simulink library "socmemlib"  (R2021a)
settings: Solver=VariableStepAuto  StartTime=0.0  StopTime=10.0  RelTol=1e-3
PreLoadFcn:
  | soc.internal.HWSWMessageTypeDef();
  | hsb.blkcb2.defineTypes;
undefined symbols (not defined in the file or in its folder): BurstRequest2BusObj, gcbh, hsb, m, ReadAccessBusObj, rearb, RegA, sendFifoFreeMsg, soc, WriteAccessBusObj
libraries: socmemlib_internal x59, priv_hsblib_beta2 x34, socsharedlib_internal x2, socqueuelib_internal x1, simulink x1
(part 1 of 5)
settings Model: Creator=The MathWorks, Inc.  LastModifiedBy=jchevali
settings SolverCC: AlgebraicLoopSolver=TrustRegion
settings DataIOCC: ReturnWorkspaceOutputs=off
settings DebuggingCC: PregeneratedLibrarySubsystemCodeDiagnostic=none  SFMachineParentedDataDiag=warning  ArithmeticOperatorsInVariantConditions=warning
settings SFSimCC: SimUseLocalCustomCode=off
settings RTWCC: RTWUseLocalCustomCode=off

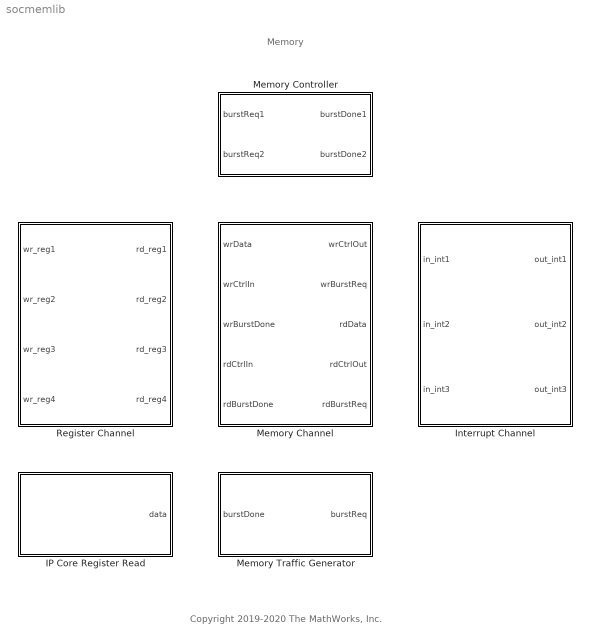
== system socmemlib ==
  note: Memory
  note: Copyright 2019-2020 The MathWorks, Inc.
  IP Core Register Read : Subsystem  InitFcn=soc.blkcb.IPCoreRegisterReadCb('InitFcnCb',gcbh);  mask(IP Core Register Read){RegisterName=RegA, OutDataTypeStr=uint16, OutputVectorSize=1, SampleTime=-1}
      mask prompts: RegisterName "Register name:"; OutDataTypeStr "Output data type:"; OutputVectorSize "Output vector size:"; SampleTime "Sample time:"
      mask help:
      | Read data from a memory-mapped register of a hardware logic IP core.
      |
      | The block interfaces with a Register Write block and outputs the read data.
      |
      | Set the Output data type and Output vector size parameters to match the equivalents in the register being read.
      mask init:
      | soc.blkcb.IPCoreRegisterReadCb('MaskInitFcn',gcbh);
      mask Help: eval('soc.internal.helpview(''soc_ipcoreregisterread'')')
      mask TypeOptions RegisterName: Variant/SIM/Wireless Read/RegisterName
      mask Callback RegisterName: soc.blkcb.IPCoreRegisterReadCb('RegisterNameCb',gcbh);
      mask TypeOptions SampleTime: Variant/SIM/Wireless Read/SampleTime
      mask DialogControl DescGroupVar Prompt: IP Core Register Read
      mask Display:
      | color('black');
      | text(0.5, 0.85, 'RegA','horizontalAlignment','center','texmode','off');
  Interrupt Channel : Subsystem  LoadFcn=soc.blkcb.InterruptChannelCb('LoadFcn', gcbh);  InitFcn=soc.blkcb.InterruptChannelCb('InitFcn', gcbh);  mask(Interrupt Channel){InterruptTable={'interrupt1','Rising edge','1';'interrupt2','Rising edge','2';'interrupt3','Rising edge','3'}, InterruptProcessingTime=100e-6, IntTableNames={'interrupt1' 'interrupt2' 'interrupt3' }, IntTableTriggers={'Rising edge' 'Rising edge' 'Rising edge' }, NumInterrupts=3, IntTableDirty=0}
      mask prompts: InterruptTable "Interrupts"; InterruptProcessingTime "Interrupt processing time:"; IntTableNames "(int table names)"; IntTableTriggers "(int table triggers)"; NumInterrupts "(num interrupts)"; IntTableDirty "(int table dirty)"
      mask help:
      | Model interrupts from FPGA to processor.
      |
      | Each pair of input and output ports with the same name represent an interrupt. On the FPGA side (HW) each input interfaces with a boolean signal from the FPGA, or an event from an Event Source or Memory Channel blocks. On the processor side (SW) each output connects to a Task Manager event input port.
      |
      | Add or remove interrupts by using the New and Delete buttons, respectively. To change the priority of interrupts, arrange their order using the Move Up and Move Down buttons. Change the Name and Trigger Type of an interrupt by editing the value in the table. Set the interrupt Trigger Type to Rising Edge if the interrupt is coming from FPGA logic. Set the interrupt Trigger Type to SoC event if the interrupt is coming from Event Source block or Memory Channel block.
      mask init:
      | soc.blkcb.InterruptChannelCb('MaskInitFcn', gcbh, gcs);
      settings: PreSaveFcn=soc.blkcb.InterruptChannelCb('PreSaveFcn', gcbh);  PreCopyFcn=soc.blkcb.InterruptChannelCb('PreCopyFcn', gcbh);
      mask Help: eval('soc.internal.helpview(''soc_interruptchannel'')')
      mask Callback InterruptTable: soc.blkcb.InterruptChannelCb('EditTableRowCb', gcbh);
      mask Callback IntTableDirty: soc.blkcb.InterruptChannelCb('ResetTableCb', gcbh);
      mask DialogControl DescGroupVar Prompt: Interrupt Channel
      mask DialogControl AddRow Prompt: New
      mask DialogControl AddRow Callback: soc.blkcb.InterruptChannelCb('AddTableRowCb', gcbh);
      mask DialogControl MoveUpRow Prompt: Move Up
      mask DialogControl MoveUpRow Callback: soc.blkcb.InterruptChannelCb('ShiftTableRowUpCb', gcbh);
      mask DialogControl MoveDownRow Prompt: Move Down
      mask DialogControl MoveDownRow Callback: soc.blkcb.InterruptChannelCb('ShiftTableRowDownCb', gcbh);
      mask DialogControl DeleteRow Prompt: Delete
      mask DialogControl DeleteRow Callback: soc.blkcb.InterruptChannelCb('DeleteTableRowCb', gcbh);
      mask DialogControl AdvancedParametersPanel Prompt: Advanced
      mask DialogControl TableSupportParameterGroup Prompt: (Parameters - hidden)
      mask Display:
      | text(0.02,0.95,'{\bfHW}','horizontalAlignment','left', 'texmode','on');
      | text(0.98,0.95,'{\bfSW}','horizontalAlignment','right','texmode','on');
      | port_label('input', 1, 'interrupt1');
      | port_label('input', 2, 'interrupt2');
      | port_label('input', 3, 'interrupt3');
      | 
      | port_label('output', 1, 'interrupt1');
      | port_label('output', 2, 'interrupt2');
      | port_label('output', 3, 'interrupt3');
  Memory Channel : Subsystem  InstantiateOnLoad=on  LoadFcn=hsb.blkcb2.MemoryChannelCbV1('LoadFcn',gcbh);  InitFcn=hsb.blkcb2.MemoryChannelCbV1('InitFcn',gcbh);  mask(Memory Channel){ChannelType=AXI4-Stream FIFO, MRBufferSize=4096, MRNumBuffers=8, BurstLengthWriterChIf=256, BurstLengthReaderChIf=256, UseValuesFromTargetHardwareResources=on, ReaderWriterUseSameValues=on, FIFODepthWriter=8, FIFODepthReader=8, FIFOAFullDepthWriter=6, FIFOAFullDepthReader=6, ICClockFrequencyWriter=100, ICClockFrequencyReader=100, ICDataWidthWriter=64, ICDataWidthReader=64, ChDimensionsWriterChIf=1024, ChTypeWriterChIf=uint32, ChFrameSampleTimeWriterChIf=1, ChBitPackedWriterChIf=off, OutSigSpecMatchesInSigSpec=on, ChDimensionsReaderChIf=1024, ChTypeWithInhReaderChIf=uint32, ChFrameSampleTimeReaderChIf=1, ChBitPackedReaderChIf=off, InsertInactivePixelClocksReaderChIf=off, FrameSizeReaderChIf=160x120p, ProtocolWriter=AXI4-Stream, ProtocolReader=AXI4-Stream, ChTypeReaderChIf=uint32, LastTargetBoard=None, Beta2Compatible=off, MRRegionSize=32768, DiagnosticLevel=No debug, MRBaseAddress=hex2dec('00010000'), UseTargetGlobalValues=off, InterruptHandlingTimeWriterChIf=10e-6, BufferEventIDWriterChIf=NOT_USED, BufferLengthReaderChIf=NOT_USED, InterruptHandlingTimeReaderChIf=10e-6, BufferEventIDReaderChIf=NOT_USED}
      mask prompts: ChannelType "soc:ui:ChannelTypePR"; MRBufferSize "soc:ui:MRBufferSizePR"; MRNumBuffers "soc:ui:MRNumBuffersPR"; BurstLengthWriterChIf "Writer:"; BurstLengthReaderChIf "Reader:"; UseValuesFromTargetHardwareResources "soc:ui:UseValuesFromTargetHardwareResourcesPR"; ReaderWriterUseSameValues "soc:ui:ReaderWriterUseSameValuesPR"; FIFODepthWriter "Writer:"; FIFODepthReader "Reader:"; FIFOAFullDepthWriter "Writer:"; FIFOAFullDepthReader "Reader:"; ICClockFrequencyWriter "Writer:"; ICClockFrequencyReader "Reader:"; ICDataWidthWriter "Writer:"; ICDataWidthReader "Reader:"; ChDimensionsWriterChIf "soc:ui:ChDimensionsPR"; ChTypeWriterChIf "soc:ui:ChTypePR"; ChFrameSampleTimeWriterChIf "soc:ui:ChFrameSampleTimePR"; ChBitPackedWriterChIf "soc:ui:ChBitPackedPR"; OutSigSpecMatchesInSigSpec "soc:ui:OutSigSpecMatchesInSigSpecPR"; ChDimensionsReaderChIf "soc:ui:ChDimensionsPR"; ChTypeWithInhReaderChIf "soc:ui:ChTypeWithInhPR"; ChFrameSampleTimeReaderChIf "soc:ui:ChFrameSampleTimePR"; ChBitPackedReaderChIf "soc:ui:ChBitPackedPR"; InsertInactivePixelClocksReaderChIf "soc:ui:InsertInactivePixelClocksPR"; FrameSizeReaderChIf "soc:ui:FrameSizePR"; ProtocolWriter "soc:ui:ProtocolPR"; ProtocolReader "soc:ui:ProtocolPR"; ChTypeReaderChIf "soc:ui:ChTypePR"; LastTargetBoard "soc:ui:LastTargetBoardPR"; Beta2Compatible "soc:ui:Beta2CompatiblePR"; MRRegionSize "soc:ui:MRRegionSizePR"; DiagnosticLevel "soc:ui:DiagnosticLevelPR"; MRBaseAddress "soc:ui:MRBaseAddressPR"; UseTargetGlobalValues "soc:ui:UseTargetGlobalValuesPR"; InterruptHandlingTimeWriterChIf "soc:ui:InterruptHandlingTimePR"; BufferEventIDWriterChIf "soc:ui:BufferEventIDPR"; BufferLengthReaderChIf "soc:ui:BufferLengthPR"; InterruptHandlingTimeReaderChIf "soc:ui:InterruptHandlingTimePR"; BufferEventIDReaderChIf "soc:ui:BufferEventIDPR"
      mask help:
      | Model memory accesses as read and write bursts.
      |
      | Data, CtrlIn and CtrlOut ports read and write data. burstReq and burstDone ports manage requests to the Memory Controller.
      |
      | Burst length, Bandwidth, FIFO depth and other parameters can be changed in the Advanced section. In the Performance tab, metrics can be visualized after running a simulation.
      mask init:
      | blkH = gcbh;
      | blkDP = hsb.blkcb2.MemoryChannelCbV1('MaskInitFcnGetDerivedInfo',blkH);
      | hsb.blkcb2.MemoryChannelCbV1('MaskInitFcnSetDerivedInfo',blkH);
      settings: CopyFcn=hsb.blkcb2.MemoryChannelCbV1('CopyFcn',gcbh);  DeleteFcn=hsb.blkcb2.MemoryChannelCbV1('DeleteFcn',gcbh);  UndoDeleteFcn=hsb.blkcb2.MemoryChannelCbV1('UndoDeleteFcn',gcbh);  PreSaveFcn=hsb.blkcb2.MemoryChannelCbV1('PreSaveFcn',gcbh);  PortSchema="{\"entries\":[{\"content\":{\"connectorPositions\":[{\"content\":{\"connectorId\":\"In1\",\"location\":{\"content\":{\"denominator\":4,\"numerator\":1},\"type\":\"ConnectorPlacement.Fraction\"}},\"type\":\"ConnectorPlacement.RectBoundaryConnectorPosition\",\"uuid\":\"4c70ce42-7c73-4e93-ae07-074aaf1a9a86\"},{\"content\":{\"connectorId\":\"In2\",\"location\":{\"content\":{\"denominator\":4,\"numerator\":2},\"type\":\"ConnectorPlacement.Fraction\"}},\"type\":\"ConnectorPlacement.RectBoundaryConnectorPosition\",\"uuid\":\"b2362bf4-8aa6-405f-91d1-9667f6c9d620\"},{\"content\":{\"connectorId\":\"Out2\",\"location\":{\"content\":{\"denominator\":6,\"numerator\":1},\"type\":\"ConnectorPlacement.Fraction\"},\"rectSide\":\"TOP\"},\"type\":\"ConnectorPlacement.RectBoundaryConnectorPosition\",\"uuid\":\"7d756ea6-45bf-43e7-b630-38b77ea0e8f5\"},{\"content\":{\"connectorId\":\"Out1\",\"location\":{\"content\":{\"denominator\":4,\"numerator\":3},\"type\":\"ConnectorPlacement.Fraction\"}},\"type\":\"ConnectorPlacement.RectBoundaryConnectorPosition\",\"uuid\":\"c5018aec-8900-4eff-a24e-86b98029d217\"},{\"content\":{\"connectorId\":\"Out3\",\"location\":{\"content\":{\"denominator\":4,\"numerator\":1},\"type\":\"ConnectorPlacement.Fraction\"},\"rectSide\":\"RIGHT\"},\"type\":\"ConnectorPlacement.RectBoundaryConnectorPosition\",\"uuid\":\"77d0fbb5-db66-42ea-8c77-7d5ac595f097\"},{\"content\":{\"connectorId\":\"In3\",\"location\":{\"content\":{\"denominator\":6,\"numerator\":2},\"type\":\"ConnectorPlacement.Fraction\"},\"rectSide\":\"TOP\"},\"type\":\"ConnectorPlacement.RectBoundaryConnectorPosition\",\"uuid\":\"87aa62bc-c370-4d37-a540-9ec95a64357e\"},{\"content\":{\"connectorId\":\"<spacer>\",\"location\":{\"content\":{\"denominator\":4,\"numerator\":4},\"type\":\"ConnectorPlacement.Fraction\"}},\"type\":\"ConnectorPlacement.RectBoundaryConnectorPosition\",\"uuid\":\"c67822ed-a56d-48ae-950d-1631e90369e8\"},{\"content\":{\"connectorId\":\"<spacer>\",\"location\":{\"content\":{\"denominator\":6,\"numerator\":3},\"type\":\"ConnectorPlacement.Fraction\"},\"rectSide\":\"TOP\"},\"type\":\"ConnectorPlacement.RectBoundaryConnectorPosition\",\"uuid\":\"003a3c20-1809-4b81-91dd-db381fae4435\"},{\"content\":{\"connectorId\":\"Out4\",\"location\":{\"content\":{\"denominator\":4,\"numerator\":2},\"type\":\"ConnectorPlacement.Fraction\"},\"rectSide\":\"RIGHT\"},\"type\":\"ConnectorPlacement.RectBoundaryConnectorPosition\",\"uuid\":\"b50bd39a-3039-4a60-9d5f-00df12594061\"},{\"content\":{\"connectorId\":\"In4\",\"location\":{\"content\":{\"denominator\":4,\"numerator\":3},\"type\":\"ConnectorPlacement.Fraction\"},\"rectSide\":\"RIGHT\"},\"type\":\"ConnectorPlacement.RectBoundaryConnectorPosition\",\"uuid\":\"5399552b-01fb-4fbb-8d3f-cf2158907ef0\"},{\"content\":{\"connectorId\":\"Out5\",\"location\":{\"content\":{\"denominator\":6,\"numerator\":4},\"type\":\"ConnectorPlacement.Fraction\"},\"rectSide\":\"TOP\"},\"type\":\"ConnectorPlacement.RectBoundaryConnectorPosition\",\"uuid\":\"a671590f-6554-46f1-a67a-ef24abb9d788\"},{\"content\":{\"connectorId\":\"In5\",\"location\":{\"content\":{\"denominator\":6,\"numerator\":5},\"type\":\"ConnectorPlacement.Fraction\"},\"rectSide\":\"TOP\"},\"type\":\"ConnectorPlacement.RectBoundaryConnectorPosition\",\"uuid\":\"e91528d7-90f4-49f4-ae0e-78ad2d58a2c8\"},{\"content\":{\"connectorId\":\"<spacer>\",\"location\":{\"content\":{\"denominator\":4,\"numerator\":4},\"type\":\"ConnectorPlacement.Fraction\"},\"rectSide\":\"RIGHT\"},\"type\":\"ConnectorPlacement.RectBoundaryConnectorPosition\",\"uuid\":\"d5ea634c-b631-4c82-af2e-3f11500a48f6\"},{\"content\":{\"connectorId\":\"<spacer>\",\"location\":{\"content\":{\"denominator\":6,\"numerator\":6},\"type\":\"ConnectorPlacement.Fraction\"},\"rectSide\":\"TOP\"},\"type\":\"ConnectorPlacement.RectBoundaryConnectorPosition\",\"uuid\":\"5a3db4f9-f85f-40af-b5ea-eb4e9a0e0ae4\"}]},\"type\":\"ConnectorPlacement.ConnectorPositionOnRectBoundary\",\"uuid\":\"116a54d8-80ad-4d58-9715-56580c2de715\"}],\"packageUris\":[\"http://schema.mathworks.com/mf0/Connector/R2020b\"],\"version\":\"1.0\"}"
      mask Help: eval('soc.internal.helpview(''soc_memorychannel'')')
      mask TypeOptions ChannelType: AXI4-Stream to Software via DMA | Software to AXI4-Stream via DMA | AXI4-Stream FIFO | AXI4-Stream Video FIFO | AXI4-Stream Video Frame Buffer | AXI4 Random Access
      mask Callback ChannelType: hsb.blkcb2.MemoryChannelCbV1('MaskParamCb','ChannelType',gcbh);
      mask Callback UseValuesFromTargetHardwareResources: hsb.blkcb2.MemoryChannelCbV1('MaskParamCb','UseValuesFromTargetHardwareResources',gcbh);
      mask Callback ReaderWriterUseSameValues: hsb.blkcb2.MemoryChannelCbV1('MaskParamCb','ReaderWriterUseSameValues',gcbh);
      mask Callback OutSigSpecMatchesInSigSpec: hsb.blkcb2.MemoryChannelCbV1('MaskParamCb','OutSigSpecMatchesInSigSpec',gcbh);
      mask Callback InsertInactivePixelClocksReaderChIf: hsb.blkcb2.MemoryChannelCbV1('MaskParamCb','InsertInactivePixelClocksReaderChIf',gcbh);
      mask TypeOptions FrameSizeReaderChIf: 160x120p | 480p SDTV (720x480p) | 576p SDTV (720x576p) | 720p HDTV (1280x720p) | 1080p HDTV (1920x1080p) | 320x240p | 640x480p | 800x600p | 1024x768p | 1280x768p | 1280x1024p | 1360x768p | 1400x1050p | 1600x1200p | 1680x1050p | 1920x1200p | 16x12p (test mode)
      mask TypeOptions ProtocolWriter: AXI4-Stream | AXI4-Stream Video | AXI4 | AXI4-Stream Software
      mask Callback ProtocolWriter: hsb.blkcb2.MemoryChannelCbV1('MaskParamCb','ProtocolWriter',gcbh);
      mask TypeOptions ProtocolReader: AXI4-Stream | AXI4-Stream Video | AXI4-Stream Video with Frame Sync | AXI4 | AXI4-Stream Software
      mask Callback ProtocolReader: hsb.blkcb2.MemoryChannelCbV1('MaskParamCb','ProtocolReader',gcbh);
      mask DialogControl DescGroupVar Prompt: Memory Channel
      mask DialogControl CurrHardwareBoardText Prompt: soc:ui:CurrHardwareBoardTextPR
      mask DialogControl CurrHardwareBoardText Tooltip: soc:ui:CurrHardwareBoardTextTT
      mask DialogControl HardwareBoardLink Prompt: None
      mask DialogControl HardwareBoardLink Tooltip: soc:ui:HardwareBoardLinkTT
      mask DialogControl HardwareBoardLink Callback: hsb.blkcb2.MemoryChannelCbV1('MaskLinkCb','HardwareBoardLink',gcbh);
      mask DialogControl ShowImplementationInfoLink Prompt: soc:ui:ShowImplementationInfoLinkPR
      mask DialogControl ShowImplementationInfoLink Tooltip: soc:ui:ShowImplementationInfoLinkTT
      mask DialogControl ShowImplementationInfoLink Callback: hsb.blkcb2.MemoryChannelCbV1('MaskLinkCb','ShowImplementationInfoLink',gcbh);
      mask DialogControl MainTab Prompt: soc:ui:MainTabPR
      mask DialogControl ChannelType Prompt: Channel type:
      mask DialogControl ChannelType Tooltip: soc:ui:ChannelTypeTT
      mask DialogControl MRRegionSizeText Prompt: Region size:  32768
      mask DialogControl MRRegionSizeText Tooltip: soc:ui:MRRegionSizeTextTT
      mask DialogControl MRBufferSize Prompt: Buffer size (bytes):
      mask DialogControl MRBufferSize Tooltip: soc:ui:MRBufferSizeTT
      mask DialogControl MRNumBuffers Prompt: Number of buffers:
      mask DialogControl MRNumBuffers Tooltip: soc:ui:MRNumBuffersTT
      mask DialogControl AdvancedParametersPanel Prompt: soc:ui:AdvancedParametersPanelPR
      mask DialogControl BurstLengthGroup Prompt: soc:ui:BurstLengthGroupPR
      mask DialogControl BurstLengthWriterChIf Tooltip: soc:ui:BurstLengthTT
      mask DialogControl BurstLengthReaderChIf Tooltip: soc:ui:BurstLengthTT
      mask DialogControl UseValuesFromTargetHardwareResources Prompt: Use hardware board settings
      mask DialogControl UseValuesFromTargetHardwareResources Tooltip: soc:ui:UseValuesFromTargetHardwareResourcesTT
      mask DialogControl ReaderWriterUseSameValues Prompt: Reader/Writer use same values
      mask DialogControl ReaderWriterUseSameValues Tooltip: soc:ui:ReaderWriterUseSameValuesTT
      mask DialogControl InterconnectGroup Prompt: soc:ui:InterconnectGroupPR
      mask DialogControl FIFODepthRowHdr Prompt: soc:ui:FIFODepthRowHdrPR
      mask DialogControl FIFODepthWriter Tooltip: codertarget:ui:FPGADesignAXIMemoryInterconnectFIFODepthToolTip
      mask DialogControl FIFODepthReader Tooltip: codertarget:ui:FPGADesignAXIMemoryInterconnectFIFODepthToolTip
      mask DialogControl FIFOAFullDepthRowHdr Prompt: soc:ui:FIFOAFullDepthRowHdrPR
      mask DialogControl FIFOAFullDepthWriter Tooltip: codertarget:ui:FPGADesignAXIMemoryInterconnectFIFOAFullDepthToolTip
      mask DialogControl FIFOAFullDepthReader Tooltip: codertarget:ui:FPGADesignAXIMemoryInterconnectFIFOAFullDepthToolTip
      mask DialogControl ICClockFrequencyRowHdr Prompt: soc:ui:ICClockFrequencyRowHdrPR
      mask DialogControl ICClockFrequencyWriter Tooltip: codertarget:ui:FPGADesignAXIMemoryInterconnectInputClockToolTip
      mask DialogControl ICClockFrequencyReader Tooltip: codertarget:ui:FPGADesignAXIMemoryInterconnectInputClockToolTip
      mask DialogControl ICDataWidthRowHdr Prompt: soc:ui:ICDataWidthRowHdrPR
      mask DialogControl ICDataWidthWriter Tooltip: codertarget:ui:FPGADesignAXIMemoryInterconnectInputDataWidthToolTip
      mask DialogControl ICDataWidthReader Tooltip: codertarget:ui:FPGADesignAXIMemoryInterconnectInputDataWidthToolTip
      mask DialogControl DataSignalAttributesTab Prompt: soc:ui:DataSignalAttributesTabPR
      mask DialogControl InputDataSpecGroup Prompt: soc:ui:InputDataSpecGroupPR
      mask DialogControl ChDimensionsWriterChIf Prompt: Dimensions:
      mask DialogControl ChDimensionsWriterChIf Tooltip: soc:ui:ChDimensionsTT
      mask DialogControl ChTypeWriterChIf Prompt: Data type:
      mask DialogControl ChTypeWriterChIf Tooltip: soc:ui:ChTypeTT
      mask DialogControl ChFrameSampleTimeWriterChIf Prompt: Sample time:
      mask DialogControl ChFrameSampleTimeWriterChIf Tooltip: soc:ui:ChFrameSampleTimeTT
      mask DialogControl ChBitPackedWriterChIf Prompt: Enable sample packing (last signal dimension as channel)
      mask DialogControl ChBitPackedWriterChIf Tooltip: soc:ui:ChBitPackedTT
      mask DialogControl OutputDataSpecGroup Prompt: soc:ui:OutputDataSpecGroupPR
      mask DialogControl OutSigSpecMatchesInSigSpec Prompt: Output data signal matches input
      mask DialogControl OutSigSpecMatchesInSigSpec Tooltip: soc:ui:OutSigSpecMatchesInSigSpecTT
      mask DialogControl ChDimensionsReaderChIf Prompt: Dimensions:
      mask DialogControl ChDimensionsReaderChIf Tooltip: soc:ui:ChDimensionsTT
      mask DialogControl ChTypeWithInhReaderChIf Prompt: Data type
      mask DialogControl ChTypeWithInhReaderChIf Tooltip: soc:ui:ChTypeWithInhTT
      mask DialogControl ChFrameSampleTimeReaderChIf Prompt: Sample time:
      mask DialogControl ChFrameSampleTimeReaderChIf Tooltip: soc:ui:ChFrameSampleTimeTT
      mask DialogControl ChBitPackedReaderChIf Prompt: Enable sample packing (last signal dimension as channel)
      mask DialogControl ChBitPackedReaderChIf Tooltip: soc:ui:ChBitPackedTT
      mask DialogControl InsertInactivePixelClocksReaderChIf Prompt: Use pixel clock sample times
      mask DialogControl InsertInactivePixelClocksReaderChIf Tooltip: soc:ui:InsertInactivePixelClocksTT
      mask DialogControl FrameSizeReaderChIf Prompt: Frame size:
      mask DialogControl FrameSizeReaderChIf Tooltip: soc:ui:FrameSizeTT
      mask DialogControl HiddenParametersPanel Prompt: soc:ui:HiddenParametersPanelPR
      mask DialogControl ProtocolWriter Prompt: Protocol
      mask DialogControl ProtocolWriter Tooltip: soc:ui:ProtocolTT
      mask DialogControl ProtocolReader Prompt: Protocol
      mask DialogControl ProtocolReader Tooltip: soc:ui:ProtocolTT
      mask DialogControl ChTypeReaderChIf Prompt: Data type:
      mask DialogControl ChTypeReaderChIf Tooltip: soc:ui:ChTypeTT
      mask DialogControl LastTargetBoard Prompt: Last used hardware board
      mask DialogControl LastTargetBoard Tooltip: soc:ui:LastTargetBoardTT
      mask DialogControl Beta2Compatible Prompt: Beta2 compatible
      mask DialogControl Beta2Compatible Tooltip: soc:ui:Beta2CompatibleTT
      mask DialogControl MRRegionSize Prompt: Region size (bytes)
      mask DialogControl DiagnosticLevel Prompt: Diagnostic level
      mask DialogControl ToDeleteParametersPanel Prompt: soc:ui:ToDeleteParametersPanelPR
      mask DialogControl MRBaseAddress Prompt: Region base address
      mask DialogControl UseTargetGlobalValues Prompt: FS use target global vals
      mask DialogControl UseTargetGlobalValues Tooltip: soc:ui:UseTargetGlobalValuesTT
      mask DialogControl ToDeleteWriterGroup Prompt: soc:ui:ToDeleteWriterGroupPR
      mask DialogControl InterruptHandlingTimeWriterChIf Prompt: Interrupt handling time
      mask DialogControl InterruptHandlingTimeWriterChIf Tooltip: soc:ui:InterruptHandlingTimeTT
      mask DialogControl BufferEventIDWriterChIf Prompt: Buffer event id
      mask DialogControl ToDeleteReaderGroup Prompt: soc:ui:ToDeleteReaderGroupPR
      mask DialogControl BufferLengthReaderChIf Prompt: Buffer length (in units of scalar data)
      mask DialogControl BufferLengthReaderChIf Tooltip: soc:ui:BufferLengthTT
      mask DialogControl InterruptHandlingTimeReaderChIf Prompt: Interrupt handling time
      mask DialogControl InterruptHandlingTimeReaderChIf Tooltip: soc:ui:InterruptHandlingTimeTT
      mask DialogControl BufferEventIDReaderChIf Prompt: Buffer event id
      mask DialogControl PerformanceTab Prompt: soc:ui:PerformanceTabPR
      mask DialogControl LaunchPerformanceAppText Prompt: soc:ui:LaunchPerformanceAppTextPR
      mask DialogControl LaunchPerformanceAppButton Prompt: soc:ui:LaunchPerformanceAppButtonPR
      mask DialogControl LaunchPerformanceAppButton Tooltip: soc:ui:LaunchPerformanceAppButtonTT
      mask DialogControl LaunchPerformanceAppButton Callback: hsb.blkcb2.MemoryChannelCbV1('MaskLinkCb','LaunchPerformanceAppButton',gcbh);
  Memory Controller : Subsystem  InstantiateOnLoad=on  LoadFcn=hsb.blkcb2.MemoryControllerCbV1('LoadFcn',gcbh);  InitFcn=hsb.blkcb2.MemoryControllerCbV1('InitFcn',gcbh);  mask(Memory Controller){NumMasters=2, ICArbitrationPolicy=Round robin, UseValuesFromTargetHardwareResources=on, ControllerFrequency=100, ControllerDataWidth=64, BandwidthDerating=2.3, WriteFirstTransferLatency=4, ReadFirstTransferLatency=5, WriteLastTransferLatency=4, ReadLastTransferLatency=1, LastTargetBoard=None, DiagnosticLevel=No debug, MAX_NUM_MASTERS=12, DDRRefreshLength=4, DDRRefreshInterval=7.8, PlotTimeResolution=100e-6}
      mask prompts: NumMasters "soc:ui:NumMastersPR"; ICArbitrationPolicy "soc:ui:ICArbitrationPolicyPR"; UseValuesFromTargetHardwareResources "soc:ui:UseValuesFromTargetHardwareResourcesPR"; ControllerFrequency "soc:ui:ControllerFrequencyPR"; ControllerDataWidth "soc:ui:ControllerDataWidthPR"; BandwidthDerating "soc:ui:BandwidthDeratingPR"; WriteFirstTransferLatency "soc:ui:WriteFirstTransferLatencyPR"; ReadFirstTransferLatency "soc:ui:ReadFirstTransferLatencyPR"; WriteLastTransferLatency "soc:ui:WriteLastTransferLatencyPR"; ReadLastTransferLatency "soc:ui:ReadLastTransferLatencyPR"; LastTargetBoard "soc:ui:LastTargetBoardPR"; DiagnosticLevel "soc:ui:DiagnosticLevelPR"; MAX_NUM_MASTERS "soc:ui:MAX_NUM_MASTERSPR"; DDRRefreshLength "soc:ui:DDRRefreshLengthPR"; DDRRefreshInterval "soc:ui:DDRRefreshIntervalPR"; PlotTimeResolution "soc:ui:PlotTimeResolutionPR"
      mask help:
      | Arbitrate memory transactions for one or more Memory Channel blocks.
      |
      | Ports burstReq and burstDone arbitrate requests from Memory Channel blocks. Set the Number of masters parameter to reflect the number of memory channels in your design.
      |
      | Interconnect arbitration, Bandwidth, and other parameters can be changed in the Advanced section. In the Performance tab, metrics can be visualized after running a simulation.
      mask init:
      | blkH = gcbh;
      | blkDP = hsb.blkcb2.MemoryControllerCbV1('MaskInitFcnGetDerivedInfo',blkH);
      | hsb.blkcb2.MemoryControllerCbV1('MaskInitFcnSetDerivedInfo',blkH);
      settings: CopyFcn=hsb.blkcb2.MemoryControllerCbV1('CopyFcn',gcbh);  DeleteFcn=hsb.blkcb2.MemoryControllerCbV1('DeleteFcn',gcbh);  UndoDeleteFcn=hsb.blkcb2.MemoryControllerCbV1('UndoDeleteFcn',gcbh);  PreSaveFcn=hsb.blkcb2.MemoryControllerCbV1('PreSaveFcn',gcbh);  PortSchema="{\"entries\":[{\"content\":{\"connectorPositions\":[{\"content\":{\"connectorId\":\"In2\",\"location\":{\"content\":{\"denominator\":6,\"numerator\":4},\"type\":\"ConnectorPlacement.Fraction\"},\"rectSide\":\"BOTTOM\"},\"type\":\"ConnectorPlacement.RectBoundaryConnectorPosition\",\"uuid\":\"af78014c-30f0-4e27-bf53-36093aacc65b\"},{\"content\":{\"connectorId\":\"In1\",\"location\":{\"content\":{\"denominator\":6,\"numerator\":1},\"type\":\"ConnectorPlacement.Fraction\"},\"rectSide\":\"BOTTOM\"},\"type\":\"ConnectorPlacement.RectBoundaryConnectorPosition\",\"uuid\":\"17d4284f-a0a1-4c67-9182-377b0455c94d\"},{\"content\":{\"connectorId\":\"<spacer>\",\"location\":{\"content\":{\"denominator\":6,\"numerator\":6},\"type\":\"ConnectorPlacement.Fraction\"},\"rectSide\":\"BOTTOM\"},\"type\":\"ConnectorPlacement.RectBoundaryConnectorPosition\",\"uuid\":\"867350af-bc29-435a-ae59-282420fb66d2\"},{\"content\":{\"connectorId\":\"<spacer>\",\"location\":{\"content\":{\"denominator\":6,\"numerator\":3},\"type\":\"ConnectorPlacement.Fraction\"},\"rectSide\":\"BOTTOM\"},\"type\":\"ConnectorPlacement.RectBoundaryConnectorPosition\",\"uuid\":\"eefbdf9e-0d95-48b1-a536-bfe9b0ed9539\"},{\"content\":{\"connectorId\":\"Out1\",\"location\":{\"content\":{\"denominator\":6,\"numerator\":2},\"type\":\"ConnectorPlacement.Fraction\"},\"rectSide\":\"BOTTOM\"},\"type\":\"ConnectorPlacement.RectBoundaryConnectorPosition\",\"uuid\":\"a64d5e6e-dc45-4684-b388-29f27a38f878\"},{\"content\":{\"connectorId\":\"Out2\",\"location\":{\"content\":{\"denominator\":6,\"numerator\":5},\"type\":\"ConnectorPlacement.Fraction\"},\"rectSide\":\"BOTTOM\"},\"type\":\"ConnectorPlacement.RectBoundaryConnectorPosition\",\"uuid\":\"cc2a1d09-69b8-4e7b-8afa-2012381f2b1d\"}]},\"type\":\"ConnectorPlacement.ConnectorPositionOnRectBoundary\",\"uuid\":\"772aec0d-99b5-4118-ad40-c8857126ecd8\"}],\"packageUris\":[\"http://schema.mathworks.com/mf0/Connector/R2020b\"],\"version\":\"1.0\"}"
      mask Help: eval('soc.internal.helpview(''soc_memorycontroller'')')
      mask Callback NumMasters: hsb.blkcb2.MemoryControllerCbV1('MaskParamCb','NumMasters',gcbh);
      mask TypeOptions ICArbitrationPolicy: Round robin | Fixed port priority
      mask Callback UseValuesFromTargetHardwareResources: hsb.blkcb2.MemoryControllerCbV1('MaskParamCb','UseValuesFromTargetHardwareResources',gcbh);
      mask DialogControl DescGroupVar Prompt: Memory Controller
      mask DialogControl CurrHardwareBoardText Prompt: soc:ui:CurrHardwareBoardTextPR
      mask DialogControl CurrHardwareBoardText Tooltip: soc:ui:CurrHardwareBoardTextTT
      mask DialogControl HardwareBoardLink Prompt: None
      mask DialogControl HardwareBoardLink Tooltip: soc:ui:HardwareBoardLinkTT
      mask DialogControl HardwareBoardLink Callback: hsb.blkcb2.MemoryControllerCbV1('MaskLinkCb','HardwareBoardLink',gcbh);
      mask DialogControl MainTab Prompt: soc:ui:MainTabPR
      mask DialogControl NumMasters Prompt: Number of masters:
      mask DialogControl NumMasters Tooltip: soc:ui:NumMastersTT
      mask DialogControl AdvancedParametersPanel Prompt: soc:ui:AdvancedParametersPanelPR
      mask DialogControl ICArbitrationPolicy Prompt: Interconnect arbitration
      mask DialogControl ICArbitrationPolicy Tooltip: soc:ui:ICArbitrationPolicyTT
      mask DialogControl UseValuesFromTargetHardwareResources Prompt: Use hardware board settings
      mask DialogControl UseValuesFromTargetHardwareResources Tooltip: soc:ui:UseValuesFromTargetHardwareResourcesTT
      mask DialogControl ControllerGroup Prompt: soc:ui:ControllerGroupPR
      mask DialogControl BandwidthRowHdr Prompt: Bandwidth:  800 MB/s
      mask DialogControl ControllerFrequency Prompt: Frequency (MHz):
      mask DialogControl ControllerFrequency Tooltip: codertarget:ui:FPGADesignAXIMemorySubsystemClockToolTip
      mask DialogControl ControllerDataWidth Prompt: Data width (bits):
      mask DialogControl ControllerDataWidth Tooltip: codertarget:ui:FPGADesignAXIMemorySubsystemDataWidthToolTip
      mask DialogControl BandwidthDerating Prompt: Bandwidth derating (%):
      mask DialogControl BandwidthDerating Tooltip: codertarget:ui:FPGADesignRefreshOverheadToolTip
      mask DialogControl ReqToFirstRowHdr Prompt: soc:ui:ReqToFirstRowHdrPR
      mask DialogControl WriteFirstTransferLatency Prompt: Write:
      mask DialogControl WriteFirstTransferLatency Tooltip: codertarget:ui:FPGADesignWriteFirstTransferLatencyToolTip
      mask DialogControl ReadFirstTransferLatency Prompt: Read:
      mask DialogControl ReadFirstTransferLatency Tooltip: codertarget:ui:FPGADesignReadFirstTransferLatencyToolTip
      mask DialogControl LastToDoneRowHdr Prompt: soc:ui:LastToDoneRowHdrPR
      mask DialogControl WriteLastTransferLatency Prompt: Write:
      mask DialogControl WriteLastTransferLatency Tooltip: codertarget:ui:FPGADesignWriteLastTransferLatencyToolTip
      mask DialogControl ReadLastTransferLatency Prompt: Read:
      mask DialogControl ReadLastTransferLatency Tooltip: codertarget:ui:FPGADesignReadLastTransferLatencyToolTip
      mask DialogControl PerformanceTab Prompt: soc:ui:PerformanceTabPR
      mask DialogControl LaunchPerformanceAppText Prompt: soc:ui:LaunchPerformanceAppTextPR
      mask DialogControl LaunchPerformanceAppButton Prompt: soc:ui:LaunchPerformanceAppButtonPR
      mask DialogControl LaunchPerformanceAppButton Tooltip: soc:ui:LaunchPerformanceAppButtonTT
      mask DialogControl LaunchPerformanceAppButton Callback: hsb.blkcb2.MemoryControllerCbV1('MaskLinkCb','LaunchPerformanceAppButton',gcbh);
      mask DialogControl HiddenParametersPanel Prompt: soc:ui:HiddenParametersPanelPR
      mask DialogControl LastTargetBoard Prompt: Last used hardware board
      mask DialogControl LastTargetBoard Tooltip: soc:ui:LastTargetBoardTT
      mask DialogControl DiagnosticLevel Prompt: Diagnostic level
      mask DialogControl MAX_NUM_MASTERS Prompt: (max num masters)
      mask DialogControl ToDeleteParametersPanel Prompt: soc:ui:ToDeleteParametersPanelPR
      mask DialogControl DDRRefreshLength Prompt: DDR refresh length (clocks)
      mask DialogControl DDRRefreshLength Tooltip: soc:ui:DDRRefreshLengthTT
      mask DialogControl DDRRefreshInterval Prompt: DDR refresh interval (us)
      mask DialogControl DDRRefreshInterval Tooltip: soc:ui:DDRRefreshIntervalTT
      mask DialogControl PlotTimeResolution Prompt: Plot time resolution:
      mask DialogControl PlotTimeResolution Tooltip: soc:ui:PlotTimeResolutionTT
      mask DialogControl PlotBWUsageBtn Prompt: soc:ui:PlotBWUsageBtnPR
      mask DialogControl PlotBWUsageBtn Callback: hsb.blkcb2.MemoryControllerCbV1('MaskLinkCb','PlotBWUsageBtn',gcbh);
      mask DialogControl PlotBurstsExecutedBtn Prompt: soc:ui:PlotBurstsExecutedBtnPR
      mask DialogControl PlotBurstsExecutedBtn Callback: hsb.blkcb2.MemoryControllerCbV1('MaskLinkCb','PlotBurstsExecutedBtn',gcbh);
      mask DialogControl PlotAvgExecTimeBtn Prompt: soc:ui:PlotAvgExecTimeBtnPR
      mask DialogControl PlotAvgExecTimeBtn Callback: hsb.blkcb2.MemoryControllerCbV1('MaskLinkCb','PlotAvgExecTimeBtn',gcbh);
      mask DialogControl PlotAvgReqToExecTimeBtn Prompt: soc:ui:PlotAvgReqToExecTimeBtnPR
      mask DialogControl PlotAvgReqToExecTimeBtn Callback: hsb.blkcb2.MemoryControllerCbV1('MaskLinkCb','PlotAvgReqToExecTimeBtn',gcbh);
  Memory Traffic Generator : Subsystem  LoadFcn=hsb.blkcb2.MemoryTrafficGeneratorCb('LoadFcn',gcbh);  InitFcn=hsb.blkcb2.MemoryTrafficGeneratorCb('InitFcn',gcbh);  VariantControl=DummyMaster_Variant  mask(Memory Traffic Generator){RequestType=Writer, TotalBurstRequests=100, BurstSize=256, TimeBetweenBursts=1e-6, AllowSimOnlyParameters=on, FirstBurstTime=10e-6, MinMaxTimeBetweenBursts=[1e-6 1e-6], WaitForDone=off, EnableAssertion=on, ControllerDataWidth=64, BurstLength=32, BurstInterAccessTimes=[1e-05 1e-06 1e-06]}
      mask prompts: RequestType "soc:ui:RequestTypePR"; TotalBurstRequests "soc:ui:TotalBurstRequestsPR"; BurstSize "soc:ui:BurstSizePR"; TimeBetweenBursts "soc:ui:TimeBetweenBurstsPR"; AllowSimOnlyParameters "soc:ui:AllowSimOnlyParametersPR"; FirstBurstTime "soc:ui:FirstBurstTimePR"; MinMaxTimeBetweenBursts "soc:ui:MinMaxTimeBetweenBurstsPR"; WaitForDone "soc:ui:WaitForDonePR"; EnableAssertion "soc:ui:EnableAssertionPR"; ControllerDataWidth "Data width"; BurstLength "soc:ui:BurstLengthPR"
      mask help:
      | Generate read or write requests to memory as a dummy master. This block can be used to model the impact that another master has on your application without explicitly designing that master.
      |
      | The block outputs memory request signals which should be connected to the burstReq and burstDone ports of a Memory Controller block. These signal lines do not transmit data.
      |
      |  The Burst length parameter is derived from the Burst size and Controller Data Width specified in the Hardware Implementation Pane.
      |
      |  In generated code, this block outputs uniformly distributed traffic request signals. In simulation, when 'Allow simulation-only parameters' is selected, this block provides more control than the generated code. Set the Random time between bursts parameter to specify the min and max values between bursts.
      mask init:
      | blkH = gcbh;
      | blkDP = hsb.blkcb2.MemoryTrafficGeneratorCb('MaskInitFcnGetDerivedInfo',blkH);
      | hsb.blkcb2.MemoryTrafficGeneratorCb('MaskInitFcnSetDerivedInfo',blkH);
      settings: CopyFcn=hsb.blkcb2.MemoryTrafficGeneratorCb('CopyFcn',gcbh);  PreSaveFcn=hsb.blkcb2.MemoryTrafficGeneratorCb('PreSaveFcn',gcbh);  PortSchema="{\"entries\":[{\"content\":{\"connectorPositions\":[{\"content\":{\"connectorId\":\"<spacer>\",\"location\":{\"content\":{\"denominator\":3,\"numerator\":3},\"type\":\"ConnectorPlacement.Fraction\"},\"rectSide\":\"TOP\"},\"type\":\"ConnectorPlacement.RectBoundaryConnectorPosition\",\"uuid\":\"183841b7-2030-48ae-a684-03b06702e361\"},{\"content\":{\"connectorId\":\"In1\",\"location\":{\"content\":{\"denominator\":3,\"numerator\":2},\"type\":\"ConnectorPlacement.Fraction\"},\"rectSide\":\"TOP\"},\"type\":\"ConnectorPlacement.RectBoundaryConnectorPosition\",\"uuid\":\"f1757017-e1d6-49ae-9e6b-fc6a126f170a\"},{\"content\":{\"connectorId\":\"Out1\",\"location\":{\"content\":{\"denominator\":3,\"numerator\":1},\"type\":\"ConnectorPlacement.Fraction\"},\"rectSide\":\"TOP\"},\"type\":\"ConnectorPlacement.RectBoundaryConnectorPosition\",\"uuid\":\"62ac83b9-7e60-4d28-a057-08f682949393\"}],\"maximumSize\":-1,\"minimumSize\":-1},\"type\":\"ConnectorPlacement.ConnectorPositionOnRectBoundary\",\"uuid\":\"fe565be3-e8dd-4450-9446-957751a1c994\"}],\"packageUris\":[\"http:\\/\\/schema.mathworks.com\\/mf0\\/Connector\\/19700101\"],\"version\":\"1.0\"}"
      mask Help: eval('soc.internal.helpview(''soc_memorytrafficgenerator'')')
      mask TypeOptions RequestType: Writer | Reader
      mask Callback BurstSize: hsb.blkcb2.MemoryTrafficGeneratorCb('MaskParamCb','BurstSize',gcbh);
      mask Callback AllowSimOnlyParameters: hsb.blkcb2.MemoryTrafficGeneratorCb('MaskParamCb','AllowSimOnlyParameters',gcbh);
      mask DialogControl DescGroupVar Prompt: Memory Traffic Generator
      mask DialogControl ParametersGroup Prompt: soc:ui:ParametersGroupPR
      mask DialogControl RequestType Prompt: Request type
      mask DialogControl RequestType Tooltip: soc:ui:RequestTypeTT
      mask DialogControl TotalBurstRequests Prompt: Total burst requests
      mask DialogControl TotalBurstRequests Tooltip: soc:ui:TotalBurstRequestsTT
      mask DialogControl BurstSize Prompt: Burst size (bytes)
      mask DialogControl BurstSize Tooltip: soc:ui:BurstSizeTT
      mask DialogControl BurstLengthText Prompt:
      | Datapath width (bits):	64
      | 	Burst length (beats):	32
      mask DialogControl BurstLengthText Tooltip: soc:ui:BurstLengthTextTT
      mask DialogControl TimeBetweenBursts Prompt: Time between bursts (s):
      mask DialogControl TimeBetweenBursts Tooltip: soc:ui:TimeBetweenBurstsTT
      mask DialogControl AllowSimOnlyParameters Prompt: Allow simulation-only parameters
      mask DialogControl AllowSimOnlyParameters Tooltip: soc:ui:AllowSimOnlyParametersTT
      mask DialogControl SimOnlyParamGroup Prompt: soc:ui:SimOnlyParamGroupPR
      mask DialogControl FirstBurstTime Prompt: First burst time:
      mask DialogControl FirstBurstTime Tooltip: soc:ui:FirstBurstTimeTT
      mask DialogControl MinMaxTimeBetweenBursts Prompt: Random time between bursts (s):
      mask DialogControl MinMaxTimeBetweenBursts Tooltip: soc:ui:MinMaxTimeBetweenBurstsTT
      mask DialogControl WaitForDone Prompt: Wait for burst done
      mask DialogControl WaitForDone Tooltip: soc:ui:WaitForDoneTT
      mask DialogControl EnableAssertion Prompt: Enable assertion
      mask DialogControl EnableAssertion Tooltip: soc:ui:EnableAssertionTT
      mask DialogControl HiddenParametersPanel Prompt: soc:ui:HiddenParametersPanelPR
      mask DialogControl ControllerDataWidth Tooltip: codertarget:ui:FPGADesignAXIMemorySubsystemDataWidthToolTip
      mask DialogControl BurstLength Prompt: Burst length
      mask DialogControl BurstLength Tooltip: soc:ui:BurstLengthTT
  Register Channel : Subsystem  LoadFcn=soc.blkcb.RegisterChannelCb('LoadFcn', gcbh);  InitFcn=soc.blkcb.RegisterChannelCb('InitFcn', gcbh);  mask(Register Channel){RegisterTable={ 'reg1', 'Read', 'uint32', '1'; 'reg2', 'Read', 'uint32', '1'; 'reg3', 'Write', 'uint32', '1'; 'reg4', 'Write', 'uint32', '1' }, SampleTime=-1, RegTableNames={'reg1' 'reg2' 'reg3' 'reg4' }, RegTableRW={'Read' 'Read' 'Write' 'Write' }, RegTableDataTypes={'uint32' 'uint32' 'uint32' 'uint32' }, RegTableVectorSizes={'1' '1' '1' '1' }, NumRegisters=4, RegTableDefaultValues={'x"0000"' 'x"0000"' 'x"0000"' 'x"0000"' }, RegTableDirty=0}
      mask prompts: RegisterTable "Registers"; SampleTime "Register write sample time:"; RegTableNames "(reg table names)"; RegTableRW "(reg table read/write)"; RegTableDataTypes "(reg table data type)"; RegTableVectorSizes "(reg table vector size)"; NumRegisters "(num registers)"; RegTableDefaultValues "(reg table default values)"; RegTableDirty "(reg table dirty)"
      mask help:
      | Model the transfer of register values between processor and FPGA.
      |
      | Each pair of input and output ports with the same name represent a register. On the FPGA side (HW) each port interfaces directly with the FPGA logic. On the processor side (SW) each port interfaces directly with a Register Read block if the register direction is configured to read, or with a Register Write block if the register direction is configured to write. Alternatively IO Data Source or IO Data Sink blocks can be used instead of Register Read or Register Write blocks when there is no processor in the system.
      |
      | Add or remove registers by using the New and Delete buttons, respectively. Arrange the order of the registers using Move Up and Move Down buttons. To change the Name, Direction, Data Type and Dimension for a register, use the Edit button. Set register Direction to Read when the processor reads from the register, or to Write when the processor writes to the register. Set register Data Type and Dimension to match the values in the Register Read or Register Write blocks.
      mask init:
      | soc.blkcb.RegisterChannelCb('MaskInitFcn', gcbh, gcs);
      settings: PreSaveFcn=soc.blkcb.RegisterChannelCb('PreSaveFcn', gcbh);  PortSchema="{\"entries\":[{\"content\":{\"connectorPositions\":[{\"content\":{\"connectorId\":\"In1\",\"location\":{\"content\":{\"denominator\":5,\"numerator\":1},\"type\":\"ConnectorPlacement.Fraction\"}},\"type\":\"ConnectorPlacement.RectBoundaryConnectorPosition\",\"uuid\":\"458508fd-78ca-4f46-b007-276204efafe5\"},{\"content\":{\"connectorId\":\"Out1\",\"location\":{\"content\":{\"denominator\":5,\"numerator\":1},\"type\":\"ConnectorPlacement.Fraction\"},\"rectSide\":\"RIGHT\"},\"type\":\"ConnectorPlacement.RectBoundaryConnectorPosition\",\"uuid\":\"09488b49-a17d-46f5-b005-ec6d5882c9d9\"},{\"content\":{\"connectorId\":\"<spacer>\",\"location\":{\"content\":{\"denominator\":5,\"numerator\":5},\"type\":\"ConnectorPlacement.Fraction\"}},\"type\":\"ConnectorPlacement.RectBoundaryConnectorPosition\",\"uuid\":\"777a63c3-1d37-4d74-aac3-0f4cf0344ec4\"},{\"content\":{\"connectorId\":\"Out4\",\"location\":{\"content\":{\"denominator\":5,\"numerator\":4},\"type\":\"ConnectorPlacement.Fraction\"}},\"type\":\"ConnectorPlacement.RectBoundaryConnectorPosition\",\"uuid\":\"077911bf-3b6c-46c1-a888-69abf1b32b08\"},{\"content\":{\"connectorId\":\"In3\",\"location\":{\"content\":{\"denominator\":5,\"numerator\":3},\"type\":\"ConnectorPlacement.Fraction\"},\"rectSide\":\"RIGHT\"},\"type\":\"ConnectorPlacement.RectBoundaryConnectorPosition\",\"uuid\":\"5f055fe5-6605-4a39-9d83-34b4e1410edb\"},{\"content\":{\"connectorId\":\"In2\",\"location\":{\"content\":{\"denominator\":5,\"numerator\":2},\"type\":\"ConnectorPlacement.Fraction\"}},\"type\":\"ConnectorPlacement.RectBoundaryConnectorPosition\",\"uuid\":\"0f0cec71-76eb-43f7-ad5d-33ebf073db1f\"},{\"content\":{\"connectorId\":\"In4\",\"location\":{\"content\":{\"denominator\":5,\"numerator\":4},\"type\":\"ConnectorPlacement.Fraction\"},\"rectSide\":\"RIGHT\"},\"type\":\"ConnectorPlacement.RectBoundaryConnectorPosition\",\"uuid\":\"88d304b3-58c3-4393-b12f-9af788c70d9c\"},{\"content\":{\"connectorId\":\"Out2\",\"location\":{\"content\":{\"denominator\":5,\"numerator\":2},\"type\":\"ConnectorPlacement.Fraction\"},\"rectSide\":\"RIGHT\"},\"type\":\"ConnectorPlacement.RectBoundaryConnectorPosition\",\"uuid\":\"a8d2b435-7508-4ba0-908c-f345aec59d58\"},{\"content\":{\"connectorId\":\"Out3\",\"location\":{\"content\":{\"denominator\":5,\"numerator\":3},\"type\":\"ConnectorPlacement.Fraction\"}},\"type\":\"ConnectorPlacement.RectBoundaryConnectorPosition\",\"uuid\":\"d4640251-e546-49c1-8de7-1ddf33655ba8\"},{\"content\":{\"connectorId\":\"<spacer>\",\"location\":{\"content\":{\"denominator\":5,\"numerator\":5},\"type\":\"ConnectorPlacement.Fraction\"},\"rectSide\":\"RIGHT\"},\"type\":\"ConnectorPlacement.RectBoundaryConnectorPosition\",\"uuid\":\"ada1a2bf-2928-4c23-9b50-7bf836152d96\"}]},\"type\":\"ConnectorPlacement.ConnectorPositionOnRectBoundary\",\"uuid\":\"218be4fa-8f46-4a89-8a90-313445b27893\"}],\"packageUris\":[\"http://schema.mathworks.com/mf0/Connector/R2020b\"],\"version\":\"1.0\"}"
      mask Help: eval('soc.internal.helpview(''soc_registerchannel'')')
      mask Callback RegTableDirty: soc.blkcb.RegisterChannelCb('ResetTableCb', gcbh);
      mask DialogControl DescGroupVar Prompt: Register Channel
      mask DialogControl ParameterGroup Prompt: Parameters
      mask DialogControl AddTableRow Prompt: New
      mask DialogControl AddTableRow Callback: soc.blkcb.RegisterChannelCb('AddTableRowCb', gcbh);
      mask DialogControl EditTableRow Prompt: Edit
      mask DialogControl EditTableRow Callback: soc.blkcb.RegisterChannelCb('EditTableRowCb', gcbh);
      mask DialogControl MoveUp Prompt: Move Up
      mask DialogControl MoveUp Callback: soc.blkcb.RegisterChannelCb('ShiftTableRowUpCb', gcbh);
      mask DialogControl MoveDown Prompt: Move Down
      mask DialogControl MoveDown Callback: soc.blkcb.RegisterChannelCb('ShiftTableRowDownCb', gcbh);
      mask DialogControl Delete Prompt: Delete
      mask DialogControl Delete Callback: soc.blkcb.RegisterChannelCb('DeleteTableRowCb', gcbh);
      mask DialogControl SampleTime Tooltip: Sample time for register access.
      mask DialogControl TableSupportParameterGroup Prompt: (Parameters - hidden)
      mask DialogControl RegTableNames Tooltip: Name of individual registers in the register bank.
      mask DialogControl RegTableRW Tooltip: Read/Write property for individual registers in register bank (cell format).
      mask DialogControl RegTableDataTypes Tooltip: Data type for individual registers in register bank (cell format).
      mask DialogControl RegTableVectorSizes Tooltip: Vector size for individual registers in register bank (cell format).
      mask Display:
      | text(0.02,0.95,'{\bfHW}','horizontalAlignment','left', 'texmode','on');
      | text(0.98,0.95,'{\bfSW}','horizontalAlignment','right','texmode','on');
      | port_label('input', 1, 'reg1');
      | port_label('input', 2, 'reg2');
      | port_label('input', 3, 'reg3');
      | port_label('input', 4, 'reg4');
      | 
      | port_label('output', 1, 'reg1');
      | port_label('output', 2, 'reg2');
      | port_label('output', 3, 'reg3');
      | port_label('output', 4, 'reg4');

== system socmemlib/IP Core Register Read ==
  Variant : Subsystem  Tag=_uses_sim_codegen_variant_  Variant=on  VariantControlMode=sim codegen switching
  data : Outport  OutDataTypeStr=OutDataTypeStr  PortDimensions=OutputVectorSize  VectorParamsAs1DForOutWhenUnconnected=off
  wires:
  Variant/1(" Data") -> data/1
